simulink model "TASK_4"  (R2018a)
settings: Solver=ode45  StartTime=0.0  StopTime=10.0  RelTol=1e-3  EnableMultiTasking=on
libraries: simulink x2
settings Model: Creator=Farhan Fuad  LastModifiedBy=ASUS
settings DataIOCC: LimitDataPoints=on  SaveFormat=Array
settings OptimizationCC: LifeSpan=inf
settings DebuggingCC: SFUnexpectedBacktrackingDiag=warning  SFNoUnconditionalDefaultTransitionDiag=warning  SFExecutionAtInitializationDiag=none
settings HardwareCC: ProdBitPerPointer=32  ProdBitPerSizeT=32  ProdBitPerPtrDiffT=32  ProdLargestAtomicFloat=None  ProdIntDivRoundTo=Undefined  ProdEndianess=Unspecified  ProdWordSize=32  ProdHWDeviceType=32-bit Generic
settings ModelReferenceCC: PropagateSignalLabelsOutOfModel=off
settings CodeAppCC: StateflowObjectComments=on
settings GRTTargetCC: TargetLangStandard=C89/C90 (ANSI)  GeneratePreprocessorConditionals=Disable all
settings ConfigComp: CovMetricSettings=dw  CovHtmlReporting=on  CovSaveCumulativeToWorkspaceVar=on  CovSaveSingleToWorkspaceVar=on  CovExternalEMLEnable=off

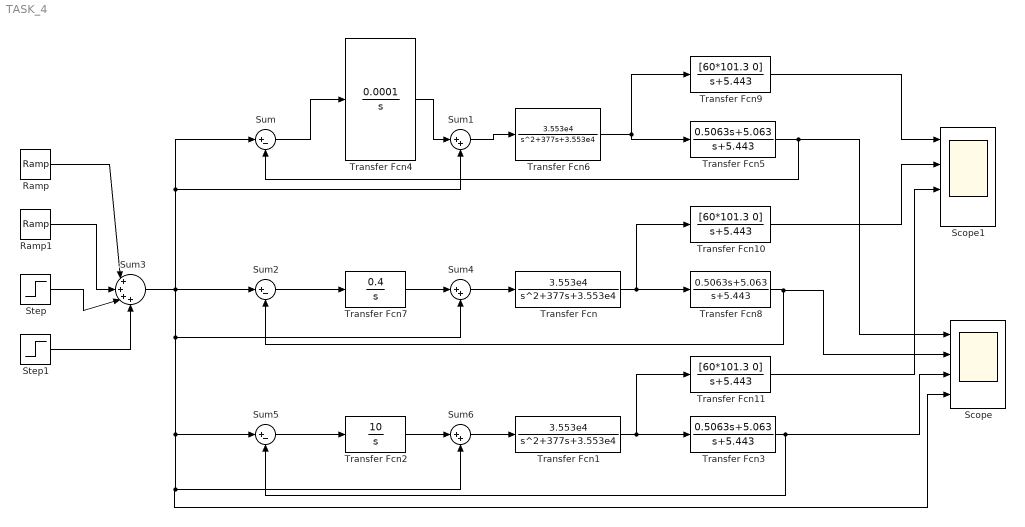
== system TASK_4 ==
  Ramp : simulink/Sources/Ramp  slope=63.158  start=1  InitialOutput=0
  Ramp1 : simulink/Sources/Ramp  slope=-63.158  start=1.23758  InitialOutput=0
  Scope : Scope  NumInputPorts=4
  Scope1 : Scope  NumInputPorts=4
  Step : Step  Time=0  After=5  SampleTime=0
  Step1 : Step  Time=5  After=-15  SampleTime=0
  Sum : Sum  Inputs=|+-
  Sum1 : Sum  Inputs=|++
  Sum2 : Sum  Inputs=|+-
  Sum3 : Sum  Inputs=|++++
  Sum4 : Sum  Inputs=|++
  Sum5 : Sum  Inputs=|+-
  Sum6 : Sum  Inputs=|++
  Transfer Fcn : TransferFcn  Numerator=[0 0 3.553e4]  Denominator=[1 377 3.553e4]
  Transfer Fcn1 : TransferFcn  Numerator=[0 0 3.553e4]  Denominator=[1 377 3.553e4]
  Transfer Fcn10 : TransferFcn  Numerator=[60*101.3 0]  Denominator=[1 5.443]
  Transfer Fcn11 : TransferFcn  Numerator=[60*101.3 0]  Denominator=[1 5.443]
  Transfer Fcn2 : TransferFcn  Numerator=[0 10]  Denominator=[1 0]
  Transfer Fcn3 : TransferFcn  Numerator=[0.5063 5.063]  Denominator=[1 5.443]
  Transfer Fcn4 : TransferFcn  Numerator=[0 0.0001]  Denominator=[1 0]
  Transfer Fcn5 : TransferFcn  Numerator=[0.5063 5.063]  Denominator=[1 5.443]
  Transfer Fcn6 : TransferFcn  Numerator=[0 0 3.553e4]  Denominator=[1 377 3.553e4]
  Transfer Fcn7 : TransferFcn  Numerator=[0 0.4]  Denominator=[1 0]
  Transfer Fcn8 : TransferFcn  Numerator=[0.5063 5.063]  Denominator=[1 5.443]
  Transfer Fcn9 : TransferFcn  Numerator=[60*101.3 0]  Denominator=[1 5.443]
  wires:
  Ramp/1 -> Sum3/1
  Step/1 -> Sum3/3
  Ramp1/1 -> Sum3/2
  Step1/1 -> Sum3/4
  Sum/1 -> Transfer Fcn4/1
  Transfer Fcn4/1 -> Sum1/1
  Sum1/1 -> Transfer Fcn6/1
  Transfer Fcn6/1 -> Transfer Fcn5/1, Transfer Fcn9/1
  Sum2/1 -> Transfer Fcn7/1
  Transfer Fcn7/1 -> Sum4/1
  Sum4/1 -> Transfer Fcn/1
  Transfer Fcn/1 -> Transfer Fcn10/1, Transfer Fcn8/1
  Sum5/1 -> Transfer Fcn2/1
  Transfer Fcn2/1 -> Sum6/1
  Sum6/1 -> Transfer Fcn1/1
  Transfer Fcn1/1 -> Transfer Fcn11/1, Transfer Fcn3/1
  Transfer Fcn9/1 -> Scope1/1
  Transfer Fcn10/1 -> Scope1/2
  Transfer Fcn11/1 -> Scope1/3
  Transfer Fcn5/1 -> Scope/1, Sum/2
  Transfer Fcn8/1 -> Scope/2, Sum2/2
  Transfer Fcn3/1 -> Scope/3, Sum5/2
  Sum3/1 -> Sum4/2, Sum5/1, Scope/4, Sum6/2, Sum2/1, Sum1/2, Sum/1
